simulink model "LPVattitudeOpenLoop"  (R2024a)
settings: Solver=VariableStepAuto  StartTime=0.0  StopTime=tf  RelTol=1e-3
values from neighbouring files (symbols this model uses):
  gamma1_initial = deg2rad(0)    [CMG_Spacecraft_Attitude_Control.m]
  gamma2_initial = deg2rad(90)    [CMG_Spacecraft_Attitude_Control.m]
libraries: simulink_extras x5, cstblocks x1
settings Model: PacingRate=1000  Creator=lanhi  LastModifiedBy=lanhi

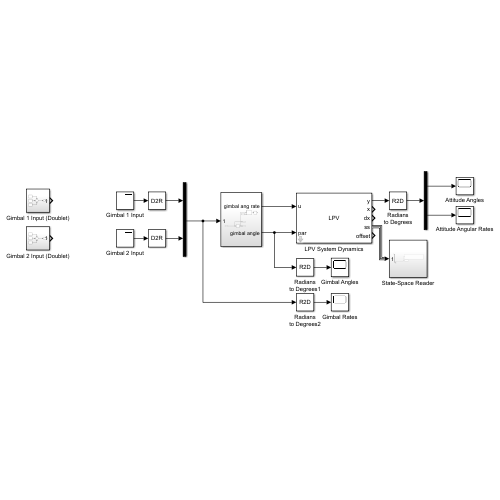
[thumbnail: Simulink's stored preview of the top-level diagram]
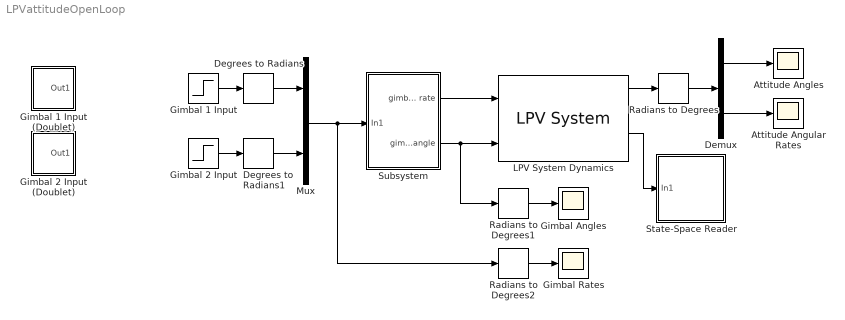
== system LPVattitudeOpenLoop ==
  Attitude Angles : Scope
  Attitude Angular Rates : Scope
  Degrees to Radians : simulink_extras/Transformations/Degrees to Radians
  Degrees to Radians1 : simulink_extras/Transformations/Degrees to Radians
  Demux : Demux  Outputs=2
  Gimbal 1 Input : Step  After=0  SampleTime=0
  Gimbal 1 Input (Doublet) : Subsystem
  Gimbal 2 Input : Step  After=0  SampleTime=0
  Gimbal 2 Input (Doublet) : Subsystem
  Gimbal Angles : Scope
  Gimbal Rates : Scope
  LPV System Dynamics : cstblocks/Linear Parameter Varying/LPV System  sys=ICs  x0=[deg2rad(15) deg2rad(12) deg2rad(8) deg2rad(0) deg2rad(0) deg2rad(0)]  opSpecOption=Specify offsets as double arrays  uOffset=0  yOffset=0  xOffset=0  opEquilOption=on  dxOffset=0  sysFixedOption=Use the first model in state-space array  sysFixed=[]  AFixed=false  BFixed=false  CFixed=false  DFixed=false  uDelayFixed=false  yDelayFixed=false  iDelayFixed=false  IMethod=Linear  EMethod=Clip  IndexSearch=Binary search  IndexBegin=on  OutputX=on  OutputXdot=on  OutputLTI=on  OutputOP=on  DataType=double  InitBufferSize=1024  FixedBuffer=off  SimMode=Interpreted execution  Offset=struct
  Mux : Mux  Inputs=2
  Radians to Degrees : simulink_extras/Transformations/Radians to Degrees
  Radians to Degrees1 : simulink_extras/Transformations/Radians to Degrees
  Radians to Degrees2 : simulink_extras/Transformations/Radians to Degrees
  State-Space Reader : Subsystem
  Subsystem : Subsystem
  wires:
  Radians to Degrees/1 -> Demux/1
  Demux/1 -> Attitude Angles/1
  Demux/2 -> Attitude Angular Rates/1
  Mux/1 -> Radians to Degrees2/1, Subsystem/1(In1)
  LPV System Dynamics/1 -> Radians to Degrees/1
  Subsystem/2(gimbal angle) -> Radians to Degrees1/1, LPV System Dynamics/2
  Radians to Degrees1/1 -> Gimbal Angles/1
  Subsystem/1(gimbal ang rate) -> LPV System Dynamics/1
  Degrees to Radians/1 -> Mux/1
  Degrees to Radians1/1 -> Mux/2
  Gimbal 1 Input/1 -> Degrees to Radians/1
  Gimbal 2 Input/1 -> Degrees to Radians1/1
  Radians to Degrees2/1 -> Gimbal Rates/1
  LPV System Dynamics/4 -> State-Space Reader/1(In1)

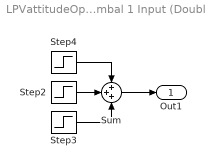
== system LPVattitudeOpenLoop/Gimbal 1 Input (Doublet) ==
  Step2 : Step  Time=5  After=-0.2  SampleTime=0
  Step3 : Step  Time=9  After=0.1  SampleTime=0
  Step4 : Step  After=0.1  SampleTime=0
  Sum : Sum  Inputs=+++
  Out1 : Outport
  wires:
  Step2/1 -> Sum/2
  Step4/1 -> Sum/1
  Step3/1 -> Sum/3
  Sum/1 -> Out1/1

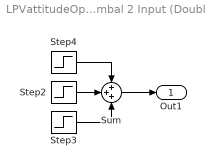
== system LPVattitudeOpenLoop/Gimbal 2 Input (Doublet) ==
  Step2 : Step  Time=5  After=-0.2  SampleTime=0
  Step3 : Step  Time=9  After=0.1  SampleTime=0
  Step4 : Step  After=0.1  SampleTime=0
  Sum : Sum  Inputs=+++
  Out1 : Outport
  wires:
  Step2/1 -> Sum/2
  Step4/1 -> Sum/1
  Step3/1 -> Sum/3
  Sum/1 -> Out1/1

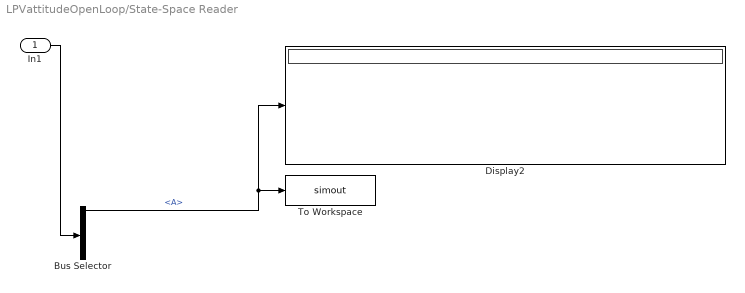
== system LPVattitudeOpenLoop/State-Space Reader ==
  In1 : Inport
  Bus Selector : BusSelector  OutputSignals=A,B,C,D
  Display2 : Display
  To Workspace : ToWorkspace  VariableName=simout  SaveFormat=Structure With Time  SampleTime=-1
  wires:
  In1/1 -> Bus Selector/1
  Bus Selector/1 -> Display2/1, To Workspace/1  "<A>"

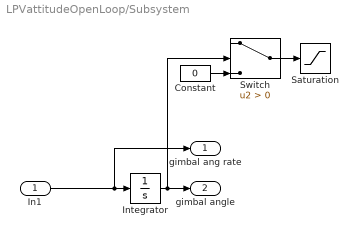
== system LPVattitudeOpenLoop/Subsystem ==
  In1 : Inport
  Constant : Constant  Value=0
  Integrator : Integrator  InitialCondition=[gamma1_initial,gamma2_initial]
  Saturation : Saturate
  Switch : Switch  Criteria=u2 > Threshold  SaturateOnIntegerOverflow=off  InputSameDT=off
  gimbal ang rate : Outport
  gimbal angle : Outport  Port=2
  wires:
  Integrator/1 -> gimbal angle/1, Switch/2
  In1/1 -> gimbal ang rate/1, Integrator/1
  Constant/1 -> Switch/3
  Switch/1 -> Saturation/1
